simulink model "position"  (R2021a)
settings: Solver=VariableStepAuto  StartTime=0.0  StopTime=inf  RelTol=1e-3
undefined symbols (not defined in the file or in its folder): aircraft
libraries: simulink x6
settings Model: Creator=DELL  LastModifiedBy=DELL

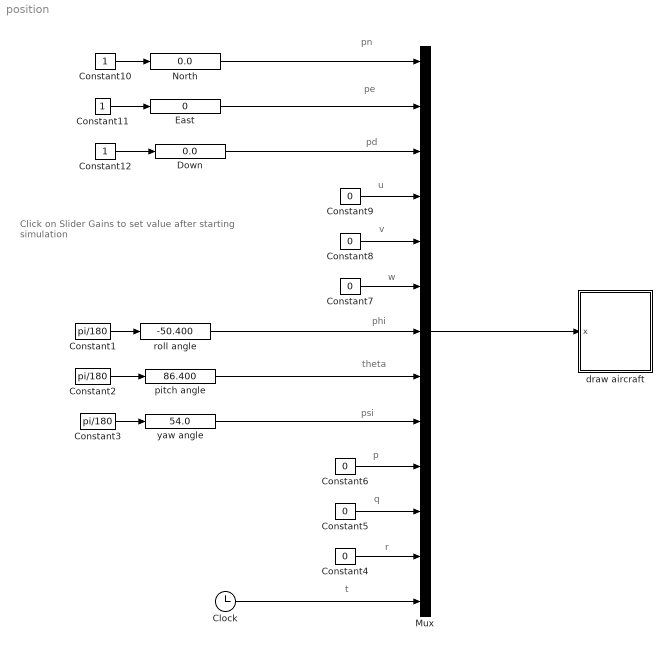
== system position ==
  note: t
  note: pn
  note: phi
  note: theta
  note: psi
  note: u
  note: r
  note: Click on Slider Gains to set value
      | after starting simulation
  note: q
  note: v
  note: pe
  note: p
  note: w
  note: pd
  Clock : Clock
  Constant1 : Constant  Value=pi/180
  Constant10 : Constant
  Constant11 : Constant
  Constant12 : Constant
  Constant2 : Constant  Value=pi/180
  Constant3 : Constant  Value=pi/180
  Constant{4..9} (6 alike) : Constant  Value=0
  Down : simulink/Math Operations/Slider Gain  gain=0.0  low=-1000  high=0
  East : simulink/Math Operations/Slider Gain  gain=0  low=-1000  high=1000
  Mux : Mux  Inputs=13
  North : simulink/Math Operations/Slider Gain  gain=0.0  low=-900  high=900
  draw aircraft : Subsystem
      mask Display: image(imread('tv.jpg'))
  pitch angle : simulink/Math Operations/Slider Gain  gain=86.400  low=-180  high=180
  roll angle : simulink/Math Operations/Slider Gain  gain=-50.400  low=-180  high=180
  "yaw angle " : simulink/Math Operations/Slider Gain  gain=54.0  low=-180  high=180
  wires:
  Constant5/1 -> Mux/11
  Down/1 -> Mux/3
  Constant12/1 -> Down/1
  Constant7/1 -> Mux/6
  East/1 -> Mux/2
  Constant6/1 -> Mux/10
  North/1 -> Mux/1
  Constant3/1 -> "yaw angle "/1
  Constant1/1 -> roll angle/1
  Constant4/1 -> Mux/12
  "yaw angle "/1 -> Mux/9
  roll angle/1 -> Mux/7
  Mux/1 -> draw aircraft/1(x)
  Constant10/1 -> North/1
  Constant9/1 -> Mux/4
  Constant8/1 -> Mux/5
  Clock/1 -> Mux/13
  Constant11/1 -> East/1
  pitch angle/1 -> Mux/8
  Constant2/1 -> pitch angle/1

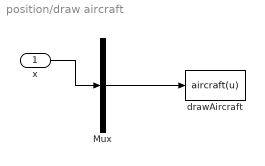
== system position/draw aircraft ==
  x : Inport
  Mux : Mux  Inputs=1
  drawAircraft : MATLABFcn  MATLABFcn=aircraft(u)  OutputDimensions=0  SampleTime=0.1
  wires:
  Mux/1 -> drawAircraft/1
  x/1 -> Mux/1
